simulink model "Supervisor_aceleracao_suave"  (R2016a)
settings: Solver=VariableStepAuto  StartTime=0.0  StopTime=10.0  RelTol=1e-3
settings Model: Creator=vmaraccini-personal  LastModifiedBy=vmaraccini-personal

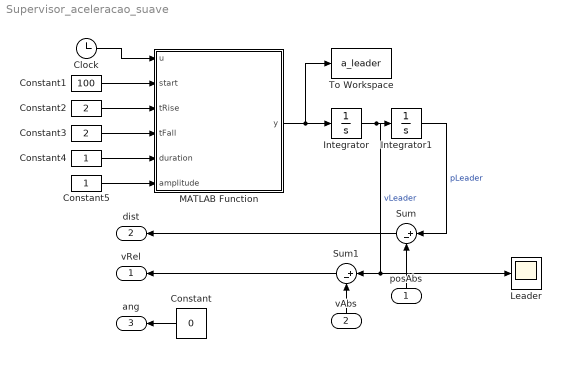
== system Supervisor_aceleracao_suave ==
  posAbs : Inport
  vAbs : Inport  Port=2
  Clock : Clock
  Constant : Constant  Value=0
  Constant1 : Constant  Value=100
  Constant2 : Constant  Value=2
  Constant3 : Constant  Value=2
  Constant4 : Constant
  Constant5 : Constant
  Integrator : Integrator  InitialCondition=13.9
  Integrator1 : Integrator  InitialCondition=40
  Leader : Scope
  MATLAB Function : MATLAB Function  TreatAsAtomicUnit=on
  Sum : Sum  Inputs=|+-
  Sum1 : Sum  Inputs=|+-
  To Workspace : ToWorkspace  VariableName=a_leader  SampleTime=-1
      settings: Save2DSignal=2-D array (concatenate along first dimension)
  vRel : Outport
  dist : Outport  Port=2
  ang : Outport  Port=3
  wires:
  Integrator1/1 -> Sum/1  "pLeader"
  Sum1/1 -> vRel/1
  vAbs/1 -> Sum1/2
  posAbs/1 -> Sum/2
  Sum/1 -> dist/1
  Integrator/1 -> Leader/1, Sum1/1, Integrator1/1  "vLeader"
  Constant/1 -> ang/1
  MATLAB Function/1(y) -> To Workspace/1, Integrator/1
  Constant1/1 -> MATLAB Function/2(start)
  Constant2/1 -> MATLAB Function/3(tRise)
  Constant3/1 -> MATLAB Function/4(tFall)
  Constant4/1 -> MATLAB Function/5(duration)
  Constant5/1 -> MATLAB Function/6(amplitude)
  Clock/1 -> MATLAB Function/1(u)

== matlab function Supervisor_aceleracao_suave/MATLAB Function ==
  data: u input; y output; start input; tRise input; tFall input; duration input; amplitude input
function y = aceleracao(u, start, tRise, tFall, duration, amplitude)
    y = (hv(u - start) - hv(u- (start+tRise) ))*amplitude.*((u-start)/tRise).^2 + ...
        (hv(u - (start+tRise)) - hv(u- (start+tRise+duration) ))*amplitude + ...
        (hv(u - (start+tRise+duration) ) - hv(u- (start+tRise+duration+tFall) ))*amplitude.*(1-((u- (start+tRise+duration) )/tFall).^2);
end

function y = hv(u)
    if u > 0
        y = 1;
    else
        y = 0;
    end
end
